simulink model "position_by_Adaptive_RBF_Attitude_by_supervised_RBFNN"  (R2015a)
settings: Solver=ode3  StartTime=0.0  StopTime=40  FixedStep=0.001  RelTol=1e-3
libraries: simulink x12, commnoisgen2 x5, dspsrcs4 x1
(part 2 of 2)

== matlab function position_by_Adaptive_RBF_Attitude_by_supervised_RBFNN/MATLAB Function7 ==
  data: y input; u input; e input; e_d input; ym output; w_1 input; w_2 input; b_1 input; b_2 input; c_1 input; c_2 input; w1 output; w2 output; b1 output; b2 output; c1 output; c2 output; o output; i input; ii output
function [ym,w1,w2,b1,b2,c1,c2,o,ii] =System(y,u,e,e_d,w_1,w_2,b_1,b_2,c_1,c_2,i)
alfa=0.07;
xite=1.9;
eta =0.0000005;
gamma=0.00000001;
K=[5.5;20;0];
E=[e;e_d];
%Lamda= [0 1 ; -30 -3]; %too slow
%Lamda= [0 1 ; -99 -25]; % vibrating
Lamda= [0 1 ; -5 -9]; %  eig(Lamda)      -0.6993  -14.3007
B=[0;1];
%Q=[0.75 0; 0 0.65];
%Q=[75 0; 0 65];
Q=[7 0; 0 5];
%P = lyap(Lamda',Q);
%P=[8.0778    0.7000;    0.7000    0.3556];
P=[    8.0778    0.7000;    0.7000    0.3556];
% alfa=0.001;
% xite=0.05;
% eta =0.005;
% gamma=0.0001;


w_1=w_1+zeros(5,1);
w_2=w_2+zeros(5,1);
b_1=b_1+zeros(5,1);
b_2=b_2+zeros(5,1);
c_1=c_1+zeros(5,1);
c_2=c_2+zeros(5,1);
if i == 0
    w=ones(5,1);
    w_1=ones(5,1);
    w_2=ones(5,1)/2;
    b=ones(5,1);
    b=[0.2; 0.2; 0.2; 0.2 ;0.2]*5; %bj
    b_1=b;
    b_2=b;
    c=ones(5,1);
    c=10*[-1.2; -0.5; 0; 0.5 ;1.2]; %cij
    c_1=c;
    c_2=c;
    
      
end

w=w_1;
w1=zeros(5,1); %%%%%%%%%%%%%%%%%%%%  W2
w2=zeros(5,1);
b=b_1;
b1=zeros(5,1);
b2=zeros(5,1);  %%%%%%%%%%%%%%%%%% b2
c=c_1;
c1=zeros(5,1);
c2=zeros(5,1);
x=u; %Input Layer
h=zeros(5,1); %hj
w=w_1;
for j=1:1:5
h(j)=exp(-norm(x-c(j))^2/(2*b(j)^2)); %Hidden Layer
end
ym=w'*h; %Output Layer

d_w=0*w;
d_w= - xite*E'*P*B*h; %%%%%%%%%%%%%%%%%%%%%%%%%%%%%%%%%%%%%%%%%%%%%%%%%%%%%%%%%%%
w = w + d_w + alfa*(w_1 - w_2);
w2 = w_1;
w1=w;

d_b=0*b;
for k=1:5
d_b(k)=(eta*(y-u))*w(k)*h(k)*(x-c(k))^2/b(k)^3;
end
b = b + d_b +gamma*(b_1 - b_2);

for k=1:5
if b(k)<= 0
    b(k)=0.1;
end
    
end
b2 = b_1;
b1=b;


d_c=0*c;
for k=1:5
d_c(k)=(eta*(y-u))*w(k)*(x-c(k))/b(k)^2;
end
c = c + d_c +gamma*(c_1 - c_2);
c2 = c_1;
c1=c;

o=u;
ii=zeros(1);
ii=i+5;

== matlab function position_by_Adaptive_RBF_Attitude_by_supervised_RBFNN/MATLAB Function8 ==
  data: G input; F_est input; phi input; theta input; zdd input; U1 output; ydd input; E input; U2 output
function [U1,U2] = fcn(G,F_est,phi,theta,zdd,ydd,E)
m=1;
g=9.81;
U1=zeros(1);
U2=zeros(1);
%K=[10;15;0];
K=[11.3;21;0];
u1= (zdd+g)*m/(cos(theta)*cos(phi));

U1=1/G*(-F_est+ydd+K'*E);
U2=K'*E;

%U1=1/G*(-F_est+K'*E);

end
% xdd = f + g u

== matlab function position_by_Adaptive_RBF_Attitude_by_supervised_RBFNN/Xdd5 ==
  data: phi input; G output; theta input; ksi input
function G = fcn(phi,theta, ksi)
m=1;
g=9.81;
G=(sin(ksi)*sin(phi)+cos(ksi)*sin(theta)*cos(phi))/m;
G=1;

== matlab function position_by_Adaptive_RBF_Attitude_by_supervised_RBFNN/Xdd6 ==
  data: fest output
function fest = fcn()

g=9.81;

fest=0;
